simulink model "lab2b"  (Simulink 7.3)
settings: Solver=FixedStepDiscrete  StartTime=0.0  StopTime=100  FixedStep=sampletime  RelTol=1e-3
libraries: dspsrcs4 x5, dspbuff3 x4, dspsnks4 x3, simulink x1
settings Model: Creator=rtadm  LastModifiedBy=freli005
settings DataIOCC: SaveOutput=off  SaveTime=off
settings OptimizationCC: BooleanDataType=off
settings DebuggingCC: SaveWithParameterizedLinksMsg=none  SignalResolutionControl=TryResolveAllWithWarning  SolverPrmCheckMsg=none  MultiTaskDSMMsg=warning  MultiTaskCondExecSysMsg=none  SFcnCompatibilityMsg=warning  StrictBusMsg=None
settings HardwareCC: TargetEndianess=LittleEndian  TargetHWDeviceType=MATLAB Host  ProdEqTarget=off
settings RTWCC: SystemTargetFile=rsim.tlc  TemplateMakefile=rsim_default_tmf  ProcessScript=rsim_make_rtw_hook  IncludeERTFirstTime=on
settings RSimTargetCC: TargetFunctionLibrary=ANSI_C  ERTMultiwordTypeDef=System defined  ERTMultiwordLength=256  IsPILTarget=off  EnableShiftOperators=on  PortableWordSizes=off

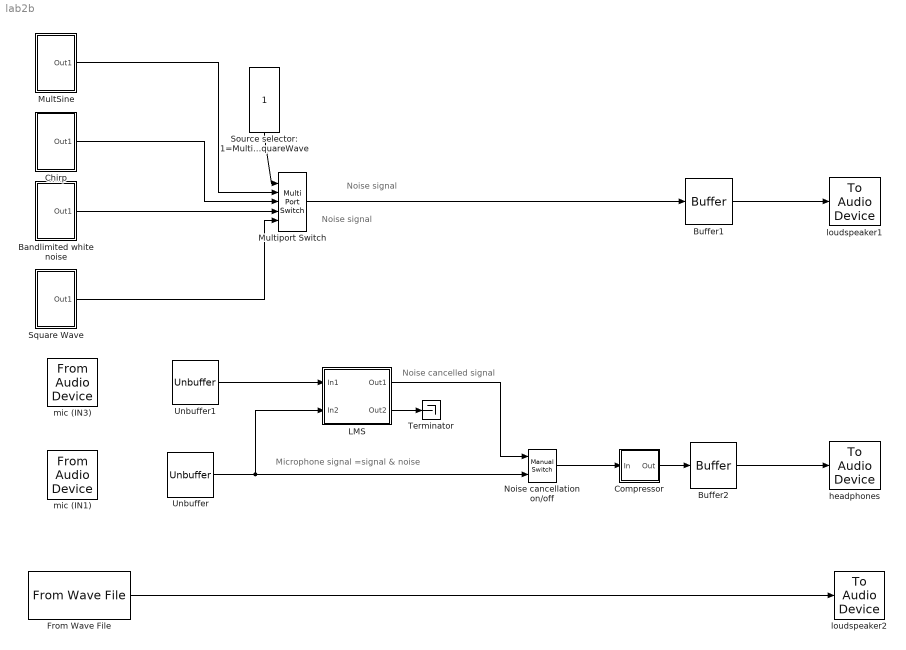
== system lab2b ==
  note: Noise cancelled signal
  note: Microphone signal
      | =signal & noise
  note: Noise signal
  note: Noise signal
  Bandlimited white noise : Subsystem
  Buffer1 : dspbuff3/Buffer  N=64  V=0  ic=0
  Buffer2 : dspbuff3/Buffer  N=64  V=0  ic=0
  Chirp : Subsystem
  Compressor : Subsystem
  From Wave File : dspsrcs4/From Wave File  FileName=nyttoljud.wav  SamplesPerFrame=4096  MinBufSize=4096  dType=double  bLoop=off  timesToPlay=1  restartMode=immediately after last sample  firstSampleOutput=off  lastSampleOutput=off
  LMS : Subsystem  mask(LMS){nnn=[1 80 20], mu=0.4, Ts=sampletime}
      mask prompts: nnn "model structure"; mu "step length"; Ts "sampletime"
      mask Display:
      | text(0.1,0.25,'y')
      | text(0.1,0.85,'u')
      | text(0.8,0.8,'eps')
      | text(0.7,0.2,'threc')
  MultSine : Subsystem
  Multiport Switch : MultiPortSwitch  Inputs=4  SaturateOnIntegerOverflow=on  InputSameDT=on
  Noise cancellation on/off : simulink/Signal Routing/Manual Switch  SystemSampleTime=-1  sw=1  action=0  varsize=off
  Source selector: 1=MultiSine 2=Chirp 3=WhiteNoise 4=SquareWave : Constant
  Square Wave : Subsystem
  Terminator : Terminator
  Unbuffer : dspbuff3/Unbuffer  ic=0
  Unbuffer1 : dspbuff3/Unbuffer  ic=0
  headphones : dspsnks4/To Audio Device  DialogController=dspDDGCreate  DialogControllerArgs=DataTag1  deviceName=3,4-INCA 88 Stereo Wave  inheritSampleRate=on  sampleRate=44100  deviceDatatype=Determine from input data type  autoBufferSize=on  bufferSize=4096  queueDuration=0.1
  loudspeaker1 : dspsnks4/To Audio Device  DialogController=dspDDGCreate  DialogControllerArgs=DataTag2  deviceName=5,6-INCA 88 Stereo Wave  inheritSampleRate=on  sampleRate=44100  deviceDatatype=Determine from input data type  autoBufferSize=on  bufferSize=4096  queueDuration=0.1
  loudspeaker2 : dspsnks4/To Audio Device  DialogController=dspDDGCreate  DialogControllerArgs=DataTag3  deviceName=7,8-INCA 88 Stereo Wave (S/PDIF, AC3, PCM)  inheritSampleRate=on  sampleRate=44100  deviceDatatype=Determine from input data type  autoBufferSize=on  bufferSize=4096  queueDuration=0.1
  mic (IN1) : dspsrcs4/From Audio Device  DialogController=dspDDGCreate  DialogControllerArgs=DataTag4  deviceName=1,2-INCA 88 Stereo Wave  numChannels=1  sampleRate=11025  deviceDatatype=Determine from output data type  autoBufferSize=on  bufferSize=4096  queueDuration=3  frameSize=64  outputDatatype=double
  mic (IN3) : dspsrcs4/From Audio Device  DialogController=dspDDGCreate  DialogControllerArgs=DataTag5  deviceName=3,4-INCA 88 Stereo Wave  numChannels=1  sampleRate=11025  deviceDatatype=Determine from output data type  autoBufferSize=on  bufferSize=4096  queueDuration=3  frameSize=64  outputDatatype=double
  wires:
  Multiport Switch/1 -> Buffer1/1
  Source selector: 1=MultiSine 2=Chirp 3=WhiteNoise 4=SquareWave/1 -> Multiport Switch/1
  MultSine/1(Out1) -> Multiport Switch/2
  Chirp/1(Out1) -> Multiport Switch/3
  Bandlimited white noise/1(Out1) -> Multiport Switch/4
  Square Wave/1(Out1) -> Multiport Switch/5
  Buffer1/1 -> loudspeaker1/1
  Buffer2/1 -> headphones/1
  Unbuffer1/1 -> LMS/1(In1)
  LMS/2(Out2) -> Terminator/1
  LMS/1(Out1) -> Noise cancellation on/off/1
  Unbuffer/1 -> LMS/2(In2), Noise cancellation on/off/2
  From Wave File/1 -> loudspeaker2/1
  Noise cancellation on/off/1 -> Compressor/1(In)
  Compressor/1(Out) -> Buffer2/1

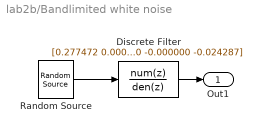
== system lab2b/Bandlimited white noise ==
  Discrete Filter : DiscreteFilter  Numerator=[0.277472 0.000000 -1.387362 0.000000 2.774724 0.000000 -2.774724 0.000000 1.387362 0.000000 -0.277472]*0.3  Denominator=[1.000000 -0.000000 -2.547368 0.000000 2.994845 -0.000000 -1.778046 0.000000 0.534570 -0.000000 -0.024287]  SampleTime=sampletime
  Random Source : dspsrcs4/Random Source  SrcType=Gaussian  NormMethod=Ziggurat  CltLength=12  MinVal=-1  MaxVal=1  MeanVal=0  VarVal=1  RepMode=Specify seed  rawSeed=1  IsInherit=off  SampMode=Discrete  SampTime=sampletime  SampFrame=1  DataType=Double  OutComplex=Real
  Out1 : Outport
  wires:
  Discrete Filter/1 -> Out1/1
  Random Source/1 -> Discrete Filter/1

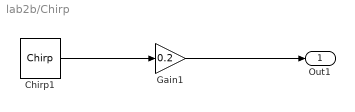
== system lab2b/Chirp ==
  Chirp1 : dspsrcs4/Chirp  sweep=Linear  mode=Bidirectional  f0=600  f1=800  t1=1  Tsweep=10  phase=0  Ts=sampletime  spf=1  datatype=Double
  Gain1 : Gain  Gain=0.2  SaturateOnIntegerOverflow=on  OutDataTypeStr=Inherit: Same as input  ParamDataTypeStr=Inherit: Same as input
  Out1 : Outport
  wires:
  Gain1/1 -> Out1/1
  Chirp1/1 -> Gain1/1

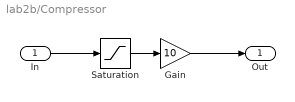
== system lab2b/Compressor ==
  In : Inport
  Gain : Gain  Gain=10  SaturateOnIntegerOverflow=on  OutDataTypeStr=Inherit: Same as input  ParamDataTypeStr=Inherit: Same as input
  Saturation : Saturate  UpperLimit=0.1  LowerLimit=-0.1
  Out : Outport
  wires:
  Saturation/1 -> Gain/1
  In/1 -> Saturation/1
  Gain/1 -> Out/1

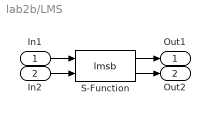
== system lab2b/LMS ==
  In1 : Inport
  In2 : Inport  Port=2
  S-Function : S-Function  FunctionName=lmsb  Parameters=nnn mu Ts  EnableBusSupport=off
  Out1 : Outport  InitialOutput=0
  Out2 : Outport  Port=2  InitialOutput=0
  wires:
  In2/1 -> S-Function/2
  S-Function/2 -> Out2/1
  In1/1 -> S-Function/1
  S-Function/1 -> Out1/1

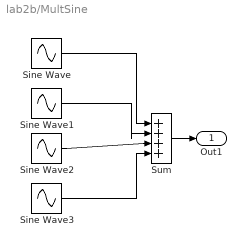
== system lab2b/MultSine ==
  Sine Wave : Sin  Amplitude=.1  Bias=0  Frequency=2*2400  Phase=0  Samples=10  SampleTime=sampletime  Offset=0
  Sine Wave1 : Sin  Amplitude=.1  Bias=0  Frequency=2*3000  Phase=0  Samples=10  SampleTime=sampletime  Offset=0
  Sine Wave2 : Sin  Amplitude=.1  Bias=0  Frequency=2*3600  Phase=0  Samples=10  SampleTime=sampletime  Offset=0
  Sine Wave3 : Sin  Amplitude=.1  Bias=0  Frequency=2*4200  Phase=0  Samples=10  SampleTime=sampletime  Offset=0
  Sum : Sum  Inputs=|++++  SaturateOnIntegerOverflow=on  InputSameDT=on  OutDataTypeStr=Inherit: Same as first input
  Out1 : Outport
  wires:
  Sine Wave/1 -> Sum/1
  Sine Wave1/1 -> Sum/2
  Sine Wave2/1 -> Sum/3
  Sine Wave3/1 -> Sum/4
  Sum/1 -> Out1/1

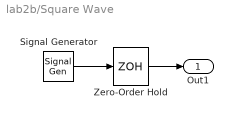
== system lab2b/Square Wave ==
  Signal Generator : SignalGenerator  WaveForm=square  Amplitude=.1  Frequency=100
  Zero-Order Hold : ZeroOrderHold  SampleTime=sampletime
  Out1 : Outport
  wires:
  Zero-Order Hold/1 -> Out1/1
  Signal Generator/1 -> Zero-Order Hold/1
